simulink model "MotorControlSim_OpenLoop"  (R2025b)
settings: Solver=ode4  StartTime=0.0  StopTime=1.5  FixedStep=1e-6  RelTol=1e-3  EnableMultiTasking=on
values from neighbouring files (symbols this model uses):
  PMSM_B = 0.000861    [MotorControlParameters.sldd]
  PMSM_J = 0.000129    [MotorControlParameters.sldd]
  Vdc = 35.0    [MotorControlParameters.sldd]
libraries: MotorControlLibrary x16, slpidlib x2
settings Model: DataDictionary=MotorControlParameters.sldd  VariantFading=off  Creator=azmib  LastModifiedBy=tka008729
settings SolverCC: ZeroCrossControl=EnableAll  AutoInsertRateTranBlk=on  MaxZcPerStep=100.0
settings DataIOCC: SaveOutput=off  SaveTime=off
settings OptimizationCC: DefaultParameterBehavior=Inlined  InlineInvariantSignals=on  EnhancedBackFolding=on  PassReuseOutputArgsAs=Individual arguments  StateBitsets=on  DataBitsets=on  ZeroExternalMemoryAtStartup=off  ZeroInternalMemoryAtStartup=off  NoFixptDivByZeroProtection=on  LifeSpan=1  OptimizeBlockOrder=speed  DifferentSizesBufferReuse=on  EfficientTunableParamExpr=on
settings DebuggingCC: SignalInfNanChecking=error  ParameterTunabilityLossMsg=error
settings HardwareCC: ProdBitPerPointer=32.0  ProdBitPerSizeT=32.0  ProdBitPerPtrDiffT=32.0  ProdLargestAtomicFloat=None  ProdIntDivRoundTo=Floor  ProdWordSize=32.0  ProdHWDeviceType=Generic->Custom
settings SFSimCC: MATLABDynamicMemAlloc=off
settings RTWCC: SystemTargetFile=ert.tlc  TLCOptions=-p0  GenCodeOnly=on  TemplateMakefile=ert_default_tmf  GenerateReport=on  RTWVerbose=off  IncludeHyperlinkInReport=on  LaunchReport=on  Description=Embedded Coder
settings CodeAppCC: ForceParamTrailComments=on  IgnoreCustomStorageClasses=off  OperatorAnnotations=on  SimulinkDataObjDesc=on  SFDataObjDesc=on  CustomSymbolStrGlobalVar=rt$N$M  CustomSymbolStrType=$N$M  CustomSymbolStrFcn=$N$M$F  CustomSymbolStrMacro=$N$M  InsertBlockDesc=on
settings ERTTargetCC: RootIOFormat=Structure reference  ERTCustomFileTemplate=example_file_process.tlc  TargetLangStandard=C99 (ISO)  CodeReplacementLibrary=ISO_C  GenerateSampleERTMain=on  IncludeMdlTerminateFcn=off  SuppressErrorStatus=on  SupportAbsoluteTime=off  PurelyIntegerCode=on  SupportNonFinite=off  SupportComplex=off
settings SimscapeCC: SimscapeNominalValues="[{\"value\":\"1\",\"unit\":\"A\"},{\"value\":\"1\",\"unit\":\"bar\"},{\"value\":\"1\",\"unit\":\"cm^2\"},{\"value\":\"1\",\"unit\":\"cm^3/s\"},{\"value\":\"1\",\"unit\":\"kJ/kg\"},{\"value\":\"1\",\"unit\":\"kW\"},{\"value\":\"1\",\"unit\":\"l\"},{\"value\":\"1\",\"unit\":\"N\"},{\"value\":\"1\",\"unit\":\"N*m\"},{\"value\":\"1\",\"unit\":\"V\"},{\"value\":\"0.001\",\"unit\":\"Wb\"}]"  SimscapeLogDataHistory=10000.0  SimscapeLogType=all

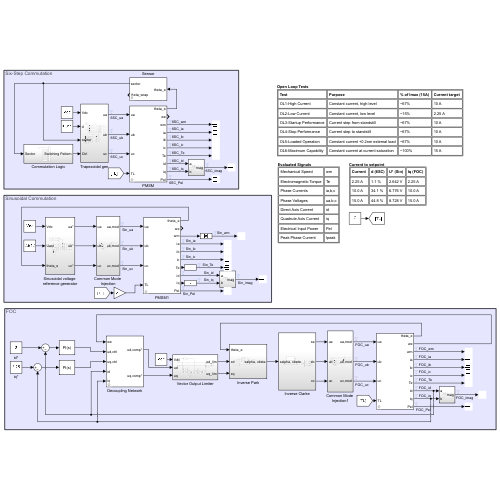
[thumbnail: Simulink's stored preview of the top-level diagram]
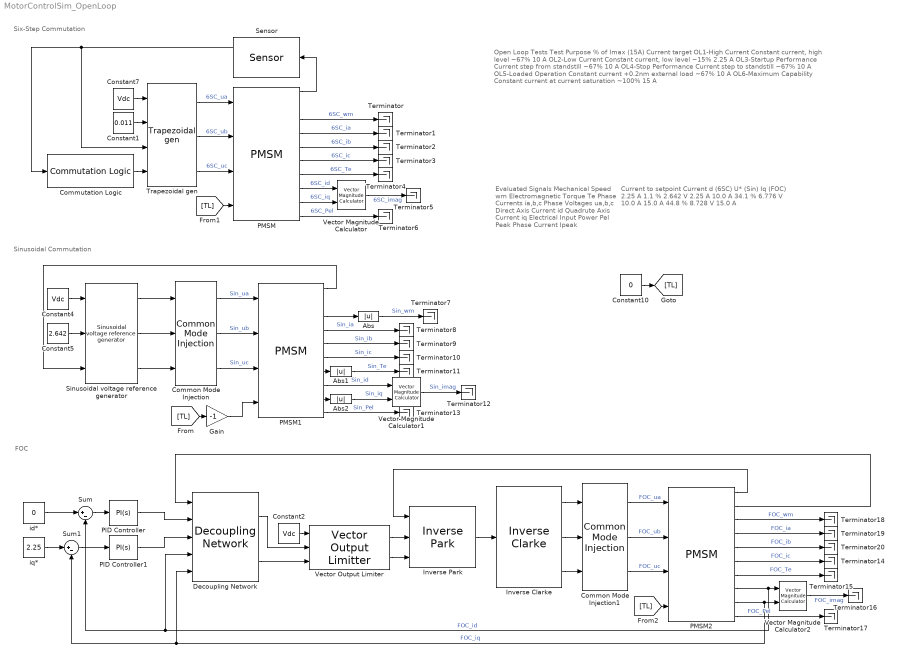
== system MotorControlSim_OpenLoop ==
  note: Evaluated Signals
      |
      | Mechanical Speed
      | wm
      |
      | Electromagnetic Torque
      | Te
      |
      | Phase Currents
      | ia,b,c
      |
      | Phase Voltages
      | ua,b,c
      |
      | Direct Axis Current
      | id
      |
      | Quadrute Axis Current
      | iq
      |
      | Electrical Input Power
      | Pel
      |
      | Peak Phase Current
      | Ipeak
  note: FOC
  note: Sinusoidal Commutation
  note: Six-Step Commutation
  note: Current to setpoint
      |
      | Current
      | d (6SC)
      | U* (Sin)
      | Iq (FOC)
      |
      | 2.25 A
      | 1.1 %
      | 2.642 V
      | 2.25 A
      |
      | 10.0 A
      | 34.1 %
      | 6.776 V
      | 10.0 A
      |
      | 15.0 A
      | 44.8 %
      | 8.728 V
      | 15.0 A
  note: Open Loop Tests
      |
      | Test
      | Purpose
      | % of Imax (15A)
      | Current target
      |
      | OL1-High Current
      | Constant current, high level
      | ~67%
      | 10 A
      |
      | OL2-Low Current
      | Constant current, low level
      | ~15%
      | 2.25 A
      |
      | OL3-Startup Performance
      | Current step from standstill
      | ~67%
      | 10 A
      |
      | OL4-Stop Performance
      | Current step to standstill
      | ~67%
      | 10 A
      |
      | OL5-Loaded Operation
      | Constant current +0.2nm external load
      | ~67%
      | 10 A
      |
      | OL6-Maximum Capability
      | Constant current at current saturation
      | ~100%
      | 15 A
  Abs : Abs  SaturateOnIntegerOverflow=off
  Abs1 : Abs  SaturateOnIntegerOverflow=off
  Abs2 : Abs  SaturateOnIntegerOverflow=off
  Common Mode Injection : MotorControlLibrary/Common Mode  Injection  SystemSampleTime=-1  VariantActivationTime=update diagram  EmptyChoice=off  PassThrough=off  PassThroughVariantControl=(default)  EmptyChoiceVariantControl=(default)  AllowFlexibleInterface=on  Latency=0  AutoFrameSizeCalculation=off
  Common Mode Injection1 : MotorControlLibrary/Common Mode  Injection  SystemSampleTime=-1  VariantActivationTime=update diagram  EmptyChoice=off  PassThrough=off  PassThroughVariantControl=(default)  EmptyChoiceVariantControl=(default)  AllowFlexibleInterface=on  Latency=0  AutoFrameSizeCalculation=off
  Commutation Logic : MotorControlLibrary/Commutation Logic  SystemSampleTime=-1  VariantActivationTime=update diagram  EmptyChoice=off  PassThrough=off  PassThroughVariantControl=(default)  EmptyChoiceVariantControl=(default)  AllowFlexibleInterface=on  Latency=0  AutoFrameSizeCalculation=off
  Constant1 : Constant  Value=0.011
  Constant10 : Constant  Value=0
  Constant2 : Constant  Value=Vdc
  Constant4 : Constant  Value=Vdc
  Constant5 : Constant  Value=2.642
  Constant7 : Constant  Value=Vdc
  Decoupling Network : MotorControlLibrary/Decoupling Network  Ls=PMSM_Ls  psi_PM=PMSM_psiPM
  Gain : Gain  Gain=-1
  Inverse Clarke : MotorControlLibrary/Inverse Clarke  SystemSampleTime=-1  VariantActivationTime=update diagram  EmptyChoice=off  PassThrough=off  PassThroughVariantControl=(default)  EmptyChoiceVariantControl=(default)  AllowFlexibleInterface=on  Latency=0  AutoFrameSizeCalculation=off
  Inverse Park : MotorControlLibrary/Inverse Park  SystemSampleTime=-1  VariantActivationTime=update diagram  EmptyChoice=off  PassThrough=off  PassThroughVariantControl=(default)  EmptyChoiceVariantControl=(default)  AllowFlexibleInterface=on  Latency=0  AutoFrameSizeCalculation=off
  PID Controller : slpidlib/PID Controller  Controller=PI  Form=Parallel  TimeDomain=Continuous-time  UseExternalTs=off  SampleTime=-1  IntegratorMethod=Forward Euler  FilterMethod=Forward Euler  ControllerParametersSource=internal  P=0.100554331907456  I=307.509314237055  UseKiTs=off  D=0  UseExternalDerivativeSource=off  N=100  UseFilter=on  TunerSelectOption=Transfer Function Based (PID Tuner App)  InitialConditionSource=internal  InitialConditionForIntegrator=0  InitialConditionForFilter=0  DifferentiatorICPrevScaledInput=0  ExternalReset=none  TrackingMode=off  Kt=1  LimitOutput=off  SatLimitsSource=internal  UpperSaturationLimit=inf  LowerSaturationLimit=-inf  LinearizeAsGain=on  AntiWindupMode=none  Kb=1  LimitIntegrator=off  UpperIntegratorSaturationLimit=inf  LowerIntegratorSaturationLimit=-inf  POutMin=[]  POutMax=[]  IOutMin=[]  IOutMax=[]  DOutMin=[]  DOutMax=[]  NOutMin=[]  NOutMax=[]  SumOutMin=[]  SumOutMax=[]  SaturationOutMin=[]  SaturationOutMax=[]  PParamMin=[]  PParamMax=[]  IParamMin=[]  IParamMax=[]  DParamMin=[]  DParamMax=[]  NParamMin=[]  NParamMax=[]  KbParamMin=[]  KbParamMax=[]  KtParamMin=[]  KtParamMax=[]  KbOutMin=[]  KbOutMax=[]  KtOutMin=[]  KtOutMax=[]  IntegratorOutMin=[]  IntegratorOutMax=[]  FilterOutMin=[]  FilterOutMax=[]  SumI1OutMin=[]  SumI1OutMax=[]  SumI2OutMin=[]  SumI2OutMax=[]  SumI3OutMin=[]  SumI3OutMax=[]  SumI4OutMin=[]  SumI4OutMax=[]  SumDOutMin=[]  SumDOutMax=[]  DifferentiatorOutMin=[]  DifferentiatorOutMax=[]  FilterDiffOutCoefMin=[]  FilterDiffOutCoefMax=[]  ReciprocalOutMin=[]  ReciprocalOutMax=[]  SumDenOutMin=[]  SumDenOutMax=[]  SumNumOutMin=[]  SumNumOutMax=[]  DivideOutMin=[]  DivideOutMax=[]  UdiffTsProdOutMin=[]  UdiffTsProdOutMax=[]  NTsProdOutMin=[]  NTsProdOutMax=[]  UintegralTsProdOutMin=[]  UintegralTsProdOutMax=[]  UngainTsProdOutMin=[]  UngainTsProdOutMax=[]  ClampingZeroOutDataTypeStr=Inherit: Inherit via back propagation  ClampingZeroOutMin=[]  ClampingZeroOutMax=[]  FilterDenConstantOutDataTypeStr=Inherit: Inherit via back propagation  FilterDenConstantOutMin=[]  FilterDenConstantOutMax=[]  PCopyOutDataTypeStr=Inherit: Inherit via back propagation  PCopyOutMin=[]  PCopyOutMax=[]  NCopyOutDataTypeStr=Inherit: Inherit via back propagation  NCopyOutMin=[]  NCopyOutMax=[]  IntegratorContinuousStateAttributes=''  IntegratorStateMustResolveToSignalObject=off  IntegratorRTWStateStorageClass=Auto  FilterContinuousStateAttributes=''  FilterStateMustResolveToSignalObject=off  FilterRTWStateStorageClass=Auto  ParallelPVariant=InternalParameters  IdealPVariant=Disabled  IVariant=InternalParameters  DVariant=Disabled  IntegratorVariant=Continuous  SatVariant=Disabled  AWVariant=Passthrough  PCopyVariant=Disabled  TRVariant=Disabled  FdbkBlocksVariant=Forward  IdealPFdbkVariant=Disabled  SatFdbkVariant=Disabled  DerivativeFilterVariant=Disabled  NVariant=Disabled  NCopyVariant=Disabled_SignalSpec  FilterICVariant=Disabled  IntegratorICVariant=InternalICs  ExternalResetVariant=Disabled  TRSumVariant=Passthrough  SumFdbkVariant=Disabled  SumVariant=Sum_PI  TsampFilterVariant=InternalTs  TsampNgainVariant=Passthrough  TsampIntegralVariant=Disabled_SignalSpec  ExternalSaturationOutDataTypeStr=Inherit: Same as second input  DerivativeSourceVariant=Disabled  PreIntVariant=InternalPreInt
  PID Controller1 : slpidlib/PID Controller  Controller=PI  Form=Parallel  TimeDomain=Continuous-time  UseExternalTs=off  SampleTime=-1  IntegratorMethod=Forward Euler  FilterMethod=Forward Euler  ControllerParametersSource=internal  P=0.0927094132460324  I=354.116719915648  UseKiTs=off  D=0  UseExternalDerivativeSource=off  N=100  UseFilter=on  TunerSelectOption=Transfer Function Based (PID Tuner App)  InitialConditionSource=internal  InitialConditionForIntegrator=0  InitialConditionForFilter=0  DifferentiatorICPrevScaledInput=0  ExternalReset=none  TrackingMode=off  Kt=1  LimitOutput=off  SatLimitsSource=internal  UpperSaturationLimit=inf  LowerSaturationLimit=-inf  LinearizeAsGain=on  AntiWindupMode=none  Kb=1  LimitIntegrator=off  UpperIntegratorSaturationLimit=inf  LowerIntegratorSaturationLimit=-inf  POutMin=[]  POutMax=[]  IOutMin=[]  IOutMax=[]  DOutMin=[]  DOutMax=[]  NOutMin=[]  NOutMax=[]  SumOutMin=[]  SumOutMax=[]  SaturationOutMin=[]  SaturationOutMax=[]  PParamMin=[]  PParamMax=[]  IParamMin=[]  IParamMax=[]  DParamMin=[]  DParamMax=[]  NParamMin=[]  NParamMax=[]  KbParamMin=[]  KbParamMax=[]  KtParamMin=[]  KtParamMax=[]  KbOutMin=[]  KbOutMax=[]  KtOutMin=[]  KtOutMax=[]  IntegratorOutMin=[]  IntegratorOutMax=[]  FilterOutMin=[]  FilterOutMax=[]  SumI1OutMin=[]  SumI1OutMax=[]  SumI2OutMin=[]  SumI2OutMax=[]  SumI3OutMin=[]  SumI3OutMax=[]  SumI4OutMin=[]  SumI4OutMax=[]  SumDOutMin=[]  SumDOutMax=[]  DifferentiatorOutMin=[]  DifferentiatorOutMax=[]  FilterDiffOutCoefMin=[]  FilterDiffOutCoefMax=[]  ReciprocalOutMin=[]  ReciprocalOutMax=[]  SumDenOutMin=[]  SumDenOutMax=[]  SumNumOutMin=[]  SumNumOutMax=[]  DivideOutMin=[]  DivideOutMax=[]  UdiffTsProdOutMin=[]  UdiffTsProdOutMax=[]  NTsProdOutMin=[]  NTsProdOutMax=[]  UintegralTsProdOutMin=[]  UintegralTsProdOutMax=[]  UngainTsProdOutMin=[]  UngainTsProdOutMax=[]  ClampingZeroOutDataTypeStr=Inherit: Inherit via back propagation  ClampingZeroOutMin=[]  ClampingZeroOutMax=[]  FilterDenConstantOutDataTypeStr=Inherit: Inherit via back propagation  FilterDenConstantOutMin=[]  FilterDenConstantOutMax=[]  PCopyOutDataTypeStr=Inherit: Inherit via back propagation  PCopyOutMin=[]  PCopyOutMax=[]  NCopyOutDataTypeStr=Inherit: Inherit via back propagation  NCopyOutMin=[]  NCopyOutMax=[]  IntegratorContinuousStateAttributes=''  IntegratorStateMustResolveToSignalObject=off  IntegratorRTWStateStorageClass=Auto  FilterContinuousStateAttributes=''  FilterStateMustResolveToSignalObject=off  FilterRTWStateStorageClass=Auto  ParallelPVariant=InternalParameters  IdealPVariant=Disabled  IVariant=InternalParameters  DVariant=Disabled  IntegratorVariant=Continuous  SatVariant=Disabled  AWVariant=Passthrough  PCopyVariant=Disabled  TRVariant=Disabled  FdbkBlocksVariant=Forward  IdealPFdbkVariant=Disabled  SatFdbkVariant=Disabled  DerivativeFilterVariant=Disabled  NVariant=Disabled  NCopyVariant=Disabled_SignalSpec  FilterICVariant=Disabled  IntegratorICVariant=InternalICs  ExternalResetVariant=Disabled  TRSumVariant=Passthrough  SumFdbkVariant=Disabled  SumVariant=Sum_PI  TsampFilterVariant=InternalTs  TsampNgainVariant=Passthrough  TsampIntegralVariant=Disabled_SignalSpec  ExternalSaturationOutDataTypeStr=Inherit: Same as second input  DerivativeSourceVariant=Disabled  PreIntVariant=InternalPreInt
  PMSM : MotorControlLibrary/PMSM  Rs=PMSM_Rs  Ls=PMSM_Ls  psi_PM=PMSM_psiPM  p=PMSM_p  J=PMSM_J  B=PMSM_B
  PMSM1 : MotorControlLibrary/PMSM  Rs=PMSM_Rs  Ls=PMSM_Ls  psi_PM=PMSM_psiPM  p=PMSM_p  J=PMSM_J  B=PMSM_B
  PMSM2 : MotorControlLibrary/PMSM  Rs=PMSM_Rs  Ls=PMSM_Ls  psi_PM=PMSM_psiPM  p=PMSM_p  J=PMSM_J  B=PMSM_B
  Sensor : MotorControlLibrary/Sensor  phi_e=150
  Sinusoidal voltage reference generator : MotorControlLibrary/Sinusoidal voltage  reference generator  SystemSampleTime=-1  VariantActivationTime=update diagram  EmptyChoice=off  PassThrough=off  PassThroughVariantControl=(default)  EmptyChoiceVariantControl=(default)  AllowFlexibleInterface=on  Latency=0  AutoFrameSizeCalculation=off
  Sum : Sum  Inputs=|+-
  Sum1 : Sum  Inputs=|+-
  Terminator{,1..20} (21 alike) : Terminator
  Trapezoidal gen : MotorControlLibrary/Trapezoidal gen  SystemSampleTime=-1  VariantActivationTime=update diagram  EmptyChoice=off  PassThrough=off  PassThroughVariantControl=(default)  EmptyChoiceVariantControl=(default)  AllowFlexibleInterface=on  Latency=0  AutoFrameSizeCalculation=off
  Vector Magnitude Calculator : MotorControlLibrary/Vector Magnitude Calculator  SystemSampleTime=-1  VariantActivationTime=update diagram  EmptyChoice=off  PassThrough=off  PassThroughVariantControl=(default)  EmptyChoiceVariantControl=(default)  AllowFlexibleInterface=on  Latency=0  AutoFrameSizeCalculation=off
  Vector Magnitude Calculator1 : MotorControlLibrary/Vector Magnitude Calculator  SystemSampleTime=-1  VariantActivationTime=update diagram  EmptyChoice=off  PassThrough=off  PassThroughVariantControl=(default)  EmptyChoiceVariantControl=(default)  AllowFlexibleInterface=on  Latency=0  AutoFrameSizeCalculation=off
  Vector Magnitude Calculator2 : MotorControlLibrary/Vector Magnitude Calculator  SystemSampleTime=-1  VariantActivationTime=update diagram  EmptyChoice=off  PassThrough=off  PassThroughVariantControl=(default)  EmptyChoiceVariantControl=(default)  AllowFlexibleInterface=on  Latency=0  AutoFrameSizeCalculation=off
  Vector Output Limiter : MotorControlLibrary/Vector Output Limitter  SystemSampleTime=-1  VariantActivationTime=update diagram  EmptyChoice=off  PassThrough=off  PassThroughVariantControl=(default)  EmptyChoiceVariantControl=(default)  AllowFlexibleInterface=on  Latency=0  AutoFrameSizeCalculation=off
  id* : Constant  Value=0
  iq* : Constant  Value=2.25
  wires:
  Sensor/1 -> Trapezoidal gen/3, Commutation Logic/1
  Trapezoidal gen/2 -> PMSM/2  "6SC_ub"
  Trapezoidal gen/1 -> PMSM/1  "6SC_ua"
  Trapezoidal gen/3 -> PMSM/3  "6SC_uc"
  Sinusoidal voltage reference generator/1 -> Common Mode Injection/1
  Sinusoidal voltage reference generator/2 -> Common Mode Injection/2
  Sinusoidal voltage reference generator/3 -> Common Mode Injection/3
  Common Mode Injection/1 -> PMSM1/1  "Sin_ua"
  Common Mode Injection/2 -> PMSM1/2  "Sin_ub"
  Common Mode Injection/3 -> PMSM1/3  "Sin_uc"
  Inverse Clarke/2 -> Common Mode Injection1/2
  Inverse Clarke/1 -> Common Mode Injection1/1
  Inverse Clarke/3 -> Common Mode Injection1/3
  Inverse Park/1 -> Inverse Clarke/1
  id*/1 -> Sum/1
  iq*/1 -> Sum1/1
  Constant7/1 -> Trapezoidal gen/1
  Common Mode Injection1/1 -> PMSM2/1  "FOC_ua"
  Common Mode Injection1/2 -> PMSM2/2  "FOC_ub"
  Common Mode Injection1/3 -> PMSM2/3  "FOC_uc"
  Sum/1 -> PID Controller/1
  Sum1/1 -> PID Controller1/1
  PID Controller/1 -> Decoupling Network/2
  PID Controller1/1 -> Decoupling Network/3
  Decoupling Network/1 -> Vector Output Limiter/2
  Decoupling Network/2 -> Vector Output Limiter/3
  Commutation Logic/1 -> Trapezoidal gen/4
  PMSM/1 -> Sensor/1
  PMSM2/1 -> Inverse Park/1
  PMSM2/2 -> Decoupling Network/1
  PMSM/7 -> Terminator4/1  "6SC_Te"
  PMSM/10 -> Terminator6/1  "6SC_Pel"
  PMSM/6 -> Terminator3/1  "6SC_ic"
  PMSM/5 -> Terminator2/1  "6SC_ib"
  PMSM/4 -> Terminator1/1  "6SC_ia"
  PMSM/3 -> Terminator/1  "6SC_wm"
  PMSM/8 -> Vector Magnitude Calculator/1  "6SC_id"
  PMSM/9 -> Vector Magnitude Calculator/2  "6SC_iq"
  Vector Magnitude Calculator/1 -> Terminator5/1  "6SC_imag"
  Constant4/1 -> Sinusoidal voltage reference generator/1
  Constant5/1 -> Sinusoidal voltage reference generator/2
  PMSM1/8 -> Vector Magnitude Calculator1/1  "Sin_id"
  PMSM1/5 -> Terminator9/1  "Sin_ib"
  PMSM1/10 -> Terminator13/1  "Sin_Pel"
  PMSM1/9 -> Abs2/1
  Vector Magnitude Calculator1/1 -> Terminator12/1  "Sin_imag"
  PMSM1/4 -> Terminator8/1  "Sin_ia"
  PMSM1/6 -> Terminator10/1  "Sin_ic"
  PMSM1/7 -> Abs1/1
  PMSM1/3 -> Abs/1
  Vector Magnitude Calculator2/1 -> Terminator16/1  "FOC_imag"
  PMSM2/4 -> Terminator19/1  "FOC_ia"
  PMSM2/7 -> Terminator15/1  "FOC_Te"
  PMSM2/8 -> Sum/2, Decoupling Network/4, Vector Magnitude Calculator2/1  "FOC_id"
  PMSM2/9 -> Sum1/2, Decoupling Network/5, Vector Magnitude Calculator2/2  "FOC_iq"
  PMSM2/10 -> Terminator17/1  "FOC_Pel"
  PMSM2/6 -> Terminator14/1  "FOC_ic"
  PMSM2/5 -> Terminator20/1  "FOC_ib"
  PMSM2/3 -> Terminator18/1  "FOC_wm"
  Constant2/1 -> Vector Output Limiter/1
  PMSM1/1 -> Sinusoidal voltage reference generator/3
  Abs/1 -> Terminator7/1  "Sin_wm"
  Constant1/1 -> Trapezoidal gen/2
  [TL] -> PMSM/4
  Gain/1 -> PMSM1/4
  [TL] -> PMSM2/4
  Constant10/1 -> [TL]
  [TL] -> Gain/1
  Vector Output Limiter/1 -> Inverse Park/2
  Vector Output Limiter/2 -> Inverse Park/3
  Abs1/1 -> Terminator11/1  "Sin_Te"
  Abs2/1 -> Vector Magnitude Calculator1/2  "Sin_iq"
